simulink model "GNU_Radio_868"  (Simulink 10.0)
settings: Solver=VariableStepAuto  StartTime=0.0  StopTime=0.1  RelTol=1e-3
libraries: dsparch4 x5, commchan3 x1, dspsrcs4 x1
settings Model: Creator=Pavel  LastModifiedBy=Pavel
settings DataIOCC: SaveFormat=Dataset  ReturnWorkspaceOutputs=on
settings OptimizationCC: LifeSpan=auto
settings DebuggingCC: UnderspecifiedInitializationDetection=Simplified  MergeDetectMultiDrivingBlocksExec=error  SFUnexpectedBacktrackingDiag=error  SFNoUnconditionalDefaultTransitionDiag=error  SFExecutionAtInitializationDiag=warning  ArithmeticOperatorsInVariantConditions=error
settings HardwareCC: ProdBitPerPointer=64  ProdBitPerSizeT=64  ProdBitPerPtrDiffT=64  ProdLargestAtomicFloat=Float  ProdIntDivRoundTo=Zero  ProdEndianess=LittleEndian  ProdWordSize=64  ProdHWDeviceType=Intel->x86-64 (Windows64)
settings ModelReferenceCC: PropagateSignalLabelsOutOfModel=on
settings SFSimCC: SimUseLocalCustomCode=on  CustomCodeUndefinedFunction=FilterOut
settings RTWCC: RTWUseLocalCustomCode=on
settings CodeAppCC: StateflowObjectComments=off
settings GRTTargetCC: TargetLangStandard=C99 (ISO)  CombineOutputUpdateFcns=on  GRTInterface=off
settings ConfigComp: CovMetricSettings=dwe  CovHtmlReporting=off  CovSaveCumulativeToWorkspaceVar=off  CovSaveSingleToWorkspaceVar=off

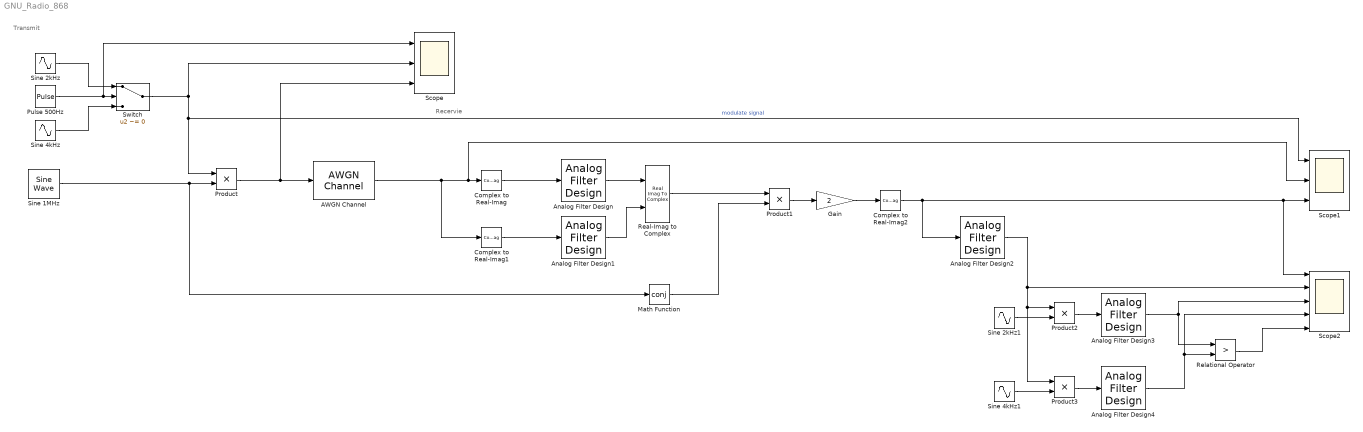
== system GNU_Radio_868 ==
  note: Recervie
  note: Transmit
  AWGN Channel : commchan3/AWGN Channel  InputProcessing=Columns as channels (frame based)  seed=67  noiseMode="Signal to noise ratio  (SNR)"  EbNodB=10  EsNodB=10  SNRdB=-10  bitsPerSym=1  Ps=1  Tsym=1  variance=1
      settings: SourceProductName=Communications Toolbox
  Analog Filter Design : dsparch4/Analog Filter Design  method=Butterworth  filttype=Bandpass  N=3  Wlo=2*pi*900e3  Whi=2*pi*1100e3  Rp=2  Rs=40
  Analog Filter Design1 : dsparch4/Analog Filter Design  method=Butterworth  filttype=Bandpass  N=3  Wlo=900e3  Whi=1100e3  Rp=2  Rs=40
  Analog Filter Design2 : dsparch4/Analog Filter Design  method=Butterworth  filttype=Lowpass  N=3  Wlo=2*pi*8e3  Whi=2*pi*1100e3  Rp=2  Rs=40
  Analog Filter Design3 : dsparch4/Analog Filter Design  method=Butterworth  filttype=Lowpass  N=3  Wlo=2*pi*1e3  Whi=2*pi*1100e3  Rp=2  Rs=40
  Analog Filter Design4 : dsparch4/Analog Filter Design  method=Butterworth  filttype=Lowpass  N=3  Wlo=2*pi*1e3  Whi=2*pi*1100e3  Rp=2  Rs=40
  Complex to Real-Imag : ComplexToRealImag  Output=Real
  Complex to Real-Imag1 : ComplexToRealImag  Output=Imag
  Complex to Real-Imag2 : ComplexToRealImag  Output=Real
  Gain : Gain  Gain=2
  Math Function : Math  Operator=conj  SignedPower=off  SaturateOnIntegerOverflow=on
  Product{,1..3} (4 alike) : Product
  Pulse 500Hz : DiscretePulseGenerator  PulseType=Time based  Period=4e-3  PulseWidth=50
  Real-Imag to Complex : RealImagToComplex
  Relational Operator : RelationalOperator  Operator=>  OutDataTypeStr=boolean  RndMeth=Simplest
  Scope : Scope  NumInputPorts=3
  Scope1 : Scope  NumInputPorts=3
  Scope2 : Scope  NumInputPorts=5
  Sine 1MHz : dspsrcs4/Sine Wave  Amplitude=1  Frequency=1e6  Phase=0  SampleMode=Discrete  OutComplex=Complex  CompMethod=Trigonometric fcn  TableSize=Speed  SampleTime=1e-7  SamplesPerFrame=1  ResetState=Restart at time zero  OutputFrames=off  dataType=double  wordLen=16  udDataType=sfix(16)  fracBitsMode=Best precision  numFracBits=15  OutDataTypeStr=double  LastOutDataTypeStr=double
  Sine 2kHz : Sin  Frequency=2*pi*2000  SampleTime=1e-6
  Sine 2kHz1 : Sin  Frequency=2*pi*2000  SampleTime=1e-6
  Sine 4kHz : Sin  Frequency=2*pi*4000  SampleTime=1e-6
  Sine 4kHz1 : Sin  Frequency=2*pi*4000  SampleTime=1e-6
  Switch : Switch  Criteria=u2 ~= 0
  wires:
  Pulse 500Hz/1 -> Scope/1, Switch/2
  Sine 2kHz/1 -> Switch/1
  Sine 4kHz/1 -> Switch/3
  Switch/1 -> Scope1/1, Product/1, Scope/2  "modulate signal"
  Sine 1MHz/1 -> Math Function/1, Product/2
  Product/1 -> Scope/3, AWGN Channel/1
  Math Function/1 -> Product1/2
  Product1/1 -> Gain/1
  AWGN Channel/1 -> Scope1/2, Complex to Real-Imag/1, Complex to Real-Imag1/1
  Complex to Real-Imag/1 -> Analog Filter Design/1
  Complex to Real-Imag1/1 -> Analog Filter Design1/1
  Analog Filter Design/1 -> Real-Imag to Complex/1
  Real-Imag to Complex/1 -> Product1/1
  Analog Filter Design1/1 -> Real-Imag to Complex/2
  Complex to Real-Imag2/1 -> Analog Filter Design2/1, Scope1/3, Scope2/1
  Analog Filter Design2/1 -> Product3/1, Product2/1, Scope2/2
  Gain/1 -> Complex to Real-Imag2/1
  Sine 4kHz1/1 -> Product3/2
  Sine 2kHz1/1 -> Product2/2
  Product2/1 -> Analog Filter Design3/1
  Product3/1 -> Analog Filter Design4/1
  Analog Filter Design4/1 -> Relational Operator/2, Scope2/4
  Analog Filter Design3/1 -> Relational Operator/1, Scope2/3
  Relational Operator/1 -> Scope2/5
